simulink model "simulador_placa"  (R2017a)
settings: Solver=FixedStepDiscrete  StartTime=0.0  StopTime=1.4  RelTol=1e-3
PreLoadFcn:
  | Ts_Power=1e-6;
  | Ts_Control=100e-6;
libraries: powerlib x2, re_lib x1
Description:
  | Copyright 2008-2017 The MathWorks, Inc.
settings Model: SimulationMode=accelerator  Creator=MathWorks  LastModifiedBy=IEEEsbUZ
settings DataIOCC: LimitDataPoints=on  SaveFormat=Array  SignalLoggingSaveFormat=ModelDataLogs  SignalLogging=off  DSMLogging=off
settings OptimizationCC: ExpressionDepthLimit=2147483647  LifeSpan=inf
settings DebuggingCC: UnderspecifiedInitializationDetection=Classic  MergeDetectMultiDrivingBlocksExec=none  SolverPrmCheckMsg=warning  FcnCallInpInsideContextMsg=warning  StateNameClashWarn=warning  SFUnexpectedBacktrackingDiag=warning  SFNoUnconditionalDefaultTransitionDiag=warning  SFExecutionAtInitializationDiag=none
settings HardwareCC: ProdBitPerPointer=32  ProdBitPerSizeT=32  ProdBitPerPtrDiffT=32  ProdLargestAtomicFloat=None  ProdIntDivRoundTo=Undefined  ProdEndianess=Unspecified  ProdWordSize=32  ProdHWDeviceType=32-bit Generic
settings ModelReferenceCC: PropagateSignalLabelsOutOfModel=off
settings GRTTargetCC: TargetLangStandard=C89/C90 (ANSI)  GeneratePreprocessorConditionals=Disable all  CombineOutputUpdateFcns=off  GRTInterface=on
settings ConfigComp: CovMetricSettings=dw  CovHtmlReporting=on  CovSaveCumulativeToWorkspaceVar=on  CovSaveSingleToWorkspaceVar=on  CovExternalEMLEnable=off  CovSFcnEnable=off

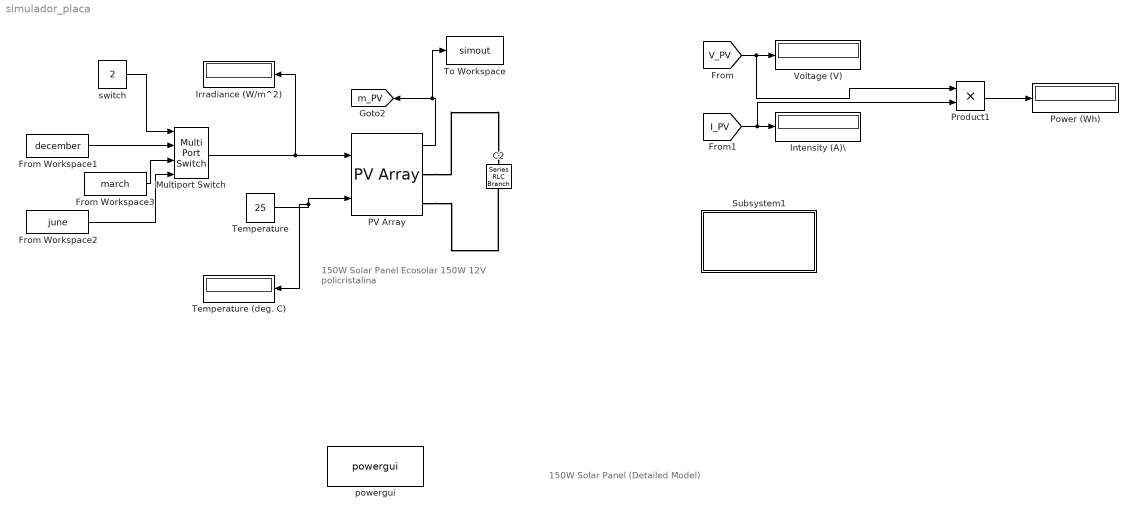
== system simulador_placa ==
  note: 150W Solar Panel (Detailed Model)
  note: 150W Solar Panel
      | Ecosolar 150W 12V policristalina
  C2 : powerlib/Elements/Series RLC Branch  LConnTagsString=__new0  RConnTagsString=__new0  BranchType=R  Resistance=2.2  Inductance=1.0  SetiL0=off  InitialCurrent=0  Capacitance=12000e-06  Setx0=off  InitialVoltage=0  Measurements=None
  From Workspace1 : FromWorkspace  VariableName=december  OutDataTypeStr=double  SampleTime=1/100000  Interpolate=off  OutputAfterFinalValue=Setting to zero
  From Workspace2 : FromWorkspace  VariableName=june  OutDataTypeStr=double  SampleTime=1/100000  Interpolate=off  OutputAfterFinalValue=Setting to zero
  "From Workspace3 " : FromWorkspace  VariableName=march  OutDataTypeStr=double  SampleTime=1/100000  Interpolate=off  OutputAfterFinalValue=Setting to zero
  Intensity (A)\ : Display
  Irradiance (W/m^2) : Display
      settings: Format=bank  Decimation=1000
  Multiport Switch : MultiPortSwitch
  PV Array : re_lib/Solar/PV Array  Npar=1  Nser=1  PlotType=array @ 1000 W/m2 & specified temperatures  S_vec="[ 1000  250 ]"  Temp_C_vec="[0 25 50  ]"  ModuleName=User-defined  PlotWhenSelected=off  Pm=149.604  Ncell=42  Voc=21.8  Isc=9.28  Vm=18.2  Im=8.22  beta_Voc_pc=-0.35119  alpha_Isc_pc=0.072921  beta_Voc=-0.076559  alpha_Isc=0.0067671  IL=9.3151  I0=2.2953e-10  nI=0.83015  Rsh=27.045  Rs=0.10231  BAL=on  Tc=Tc  Tfilter=5e-5
  Power (Wh) : Display
  Product1 : Product
  Subsystem1 : Subsystem
      mask Display: disp('Open this block\nto display additional \nscopes & measurements')
  "Temperature " : Constant  Value=25
  Temperature (deg. C) : Display
      settings: Format=bank  Decimation=1000
  To Workspace : ToWorkspace  VariableName=simout  SaveFormat=Structure  SampleTime=-1
      settings: Save2DSignal=2-D array (concatenate along first dimension)
  Voltage (V) : Display
      settings: Decimation=200
  powergui : powerlib/powergui  Priority=1  SimulationMode=Discrete  SampleTime=1e-06  frequency=60  Iterations=50  frequencyindice=0  Pbase=100e6  ErrMax=1e-4  UnitsV=kV  UnitsW=MW  buscounter=0  FunctionMessages=off  echomessages=off  EnableUseOfTLC=off  CurrentSourceSwitches=off  DisableSnubberDevices=off  DisableRonSwitches=off  DisableVfSwitches=off  DisplayEquations=off  SolverType=Tustin/Backward Euler (TBE)  Interpol=off  ExternalGateDelay=off  methode=off  Ts=0  x0status=blocks  SPID=off  SwTol=0  HookPort=off  RestoreLinks=warning  ResistiveCurrentMeasurement=off  Frange=[0:2:500]  Ylog=off  Xlog=on  ShowGrid=off  save=off  variable=ZData  structure=0  ZoomFFT=on  StartTime=0.0  cycles=1  DisplayStyle=1  fundamental=60  FreqAxis=off  MaxFrequency=1000  frequencyindicesteady=1  RmsSteady=1  display=off
  "switch " : Constant  Value=2
  tag scope: m_PV=global
  wires:
  PV Array/1 -> To Workspace/1, [m_PV]
  [I_PV] -> Product1/2, Intensity (A)\/1
  Product1/1 -> Power (Wh)/1
  "Temperature "/1 -> Temperature (deg. C)/1, PV Array/2
  Multiport Switch/1 -> Irradiance (W/m^2)/1, PV Array/1
  "From Workspace3 "/1 -> Multiport Switch/3
  From Workspace2/1 -> Multiport Switch/4
  From Workspace1/1 -> Multiport Switch/2
  "switch "/1 -> Multiport Switch/1
  [V_PV] -> Product1/1, Voltage (V)/1
  connections:
  PV Array/RConn2 -- C2/RConn1
  PV Array/RConn1 -- C2/LConn1

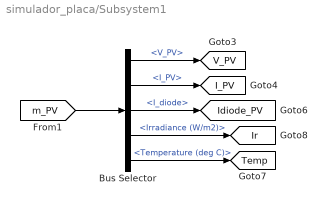
== system simulador_placa/Subsystem1 ==
  Bus Selector : BusSelector  OutputSignals=V_PV,I_PV,I_diode,Irradiance (W/m2),Temperature (deg C)
  tag scope: I_PV=global, Idiode_PV=global, Ir=global, Temp=global, V_PV=global
  wires:
  [m_PV] -> Bus Selector/1
  Bus Selector/1 -> [V_PV]  "<V_PV>"
  Bus Selector/2 -> [I_PV]  "<I_PV>"
  Bus Selector/4 -> [Ir]  "<Irradiance (W/m2)>"
  Bus Selector/3 -> [Idiode_PV]  "<I_diode>"
  Bus Selector/5 -> [Temp]  "<Temperature (deg C)>"
